simulink model "UUV_Nonlinear_Dynamic_Inversion"  (R2019b)
settings: Solver=ode45  StartTime=0.0  StopTime=600  RelTol=1e-3
undefined symbols (not defined in the file): Amp, Freq
libraries: simulink x4
settings Model: Creator=7385281  LastModifiedBy=7385281
settings SolverCC: AlgebraicLoopSolver=LineSearch

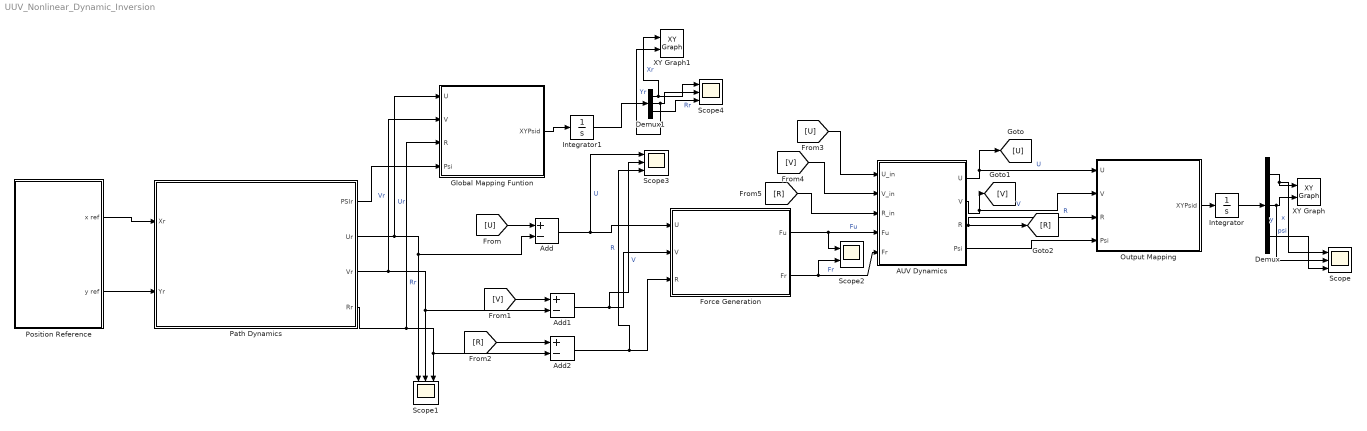
== system UUV_Nonlinear_Dynamic_Inversion ==
  AUV Dynamics : Subsystem
  Add : Sum  Inputs=+-
  Add1 : Sum  Inputs=+-
  Add2 : Sum  Inputs=+-
  Demux : Demux  Outputs=3
  Demux1 : Demux  Outputs=3
  Force Generation : Subsystem
  Global Mapping Funtion : MATLAB Function  TreatAsAtomicUnit=on
  Integrator : Integrator
  Integrator1 : Integrator
  Output Mapping : MATLAB Function  TreatAsAtomicUnit=on
  Path Dynamics : Subsystem
  Position Reference : Subsystem
  Scope{,1,3..4} (4 alike) : Scope  NumInputPorts=3
  Scope2 : Scope  NumInputPorts=2
  XY Graph : simulink/Sinks/XY Graph  xmin=-15  xmax=15  ymin=-15  ymax=15  st=-1
  XY Graph1 : simulink/Sinks/XY Graph  xmin=-15  xmax=15  ymin=-15  ymax=15  st=-1
  wires:
  Position Reference/1(x ref) -> Path Dynamics/1(Xr)
  Position Reference/2(y ref) -> Path Dynamics/2(Yr)
  Force Generation/1(Fu) -> AUV Dynamics/4(Fu), Scope2/1  "Fu"
  Force Generation/2(Fr) -> Scope2/2, AUV Dynamics/5(Fr)  "Fr"
  Path Dynamics/3(Vr) -> Global Mapping Funtion/2(V), Add1/2, Scope1/2  "Vr"
  Path Dynamics/4(Rr) -> Global Mapping Funtion/3(R), Add2/2, Scope1/3  "Rr"
  AUV Dynamics/2(V) -> Output Mapping/2(V), [V]  "V"
  AUV Dynamics/1(U) -> Output Mapping/1(U), [U]  "U"
  AUV Dynamics/3(R) -> [R], Output Mapping/3(R)  "R"
  Path Dynamics/2(Ur) -> Global Mapping Funtion/1(U), Add/2, Scope1/1  "Ur"
  [U] -> Add/1
  Add/1 -> Scope3/1, Force Generation/1(U)  "U"
  [V] -> Add1/1
  [R] -> Add2/1
  Add1/1 -> Scope3/2, Force Generation/2(V)  "V"
  Add2/1 -> Scope3/3, Force Generation/3(R)  "R"
  AUV Dynamics/4(Psi) -> Output Mapping/4(Psi)
  Output Mapping/1(XYPsid) -> Integrator/1
  Demux/1 -> Scope/1, XY Graph/1  "x"
  Demux/2 -> Scope/2, XY Graph/2  "y"
  Integrator/1 -> Demux/1
  Demux/3 -> Scope/3  "psi"
  Path Dynamics/1(PSIr) -> Global Mapping Funtion/4(Psi)
  Global Mapping Funtion/1(XYPsid) -> Integrator1/1
  Integrator1/1 -> Demux1/1
  Demux1/3 -> Scope4/3  "Rr"
  Demux1/2 -> XY Graph1/2, Scope4/2  "Yr"
  Demux1/1 -> XY Graph1/1, Scope4/1  "Xr"
  [U] -> AUV Dynamics/1(U_in)
  [V] -> AUV Dynamics/2(V_in)
  [R] -> AUV Dynamics/3(R_in)

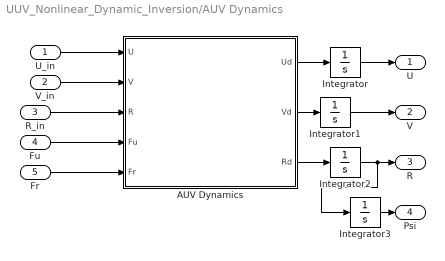
== system UUV_Nonlinear_Dynamic_Inversion/AUV Dynamics ==
  U_in : Inport
  V_in : Inport  Port=2
  R_in : Inport  Port=3
  Fu : Inport  Port=4
  Fr : Inport  Port=5
  AUV Dynamics : MATLAB Function  TreatAsAtomicUnit=on
  Integrator{,1..3} (4 alike) : Integrator
  U : Outport
  V : Outport  Port=2
  R : Outport  Port=3
  Psi : Outport  Port=4
  wires:
  Fr/1 -> AUV Dynamics/5(Fr)
  V_in/1 -> AUV Dynamics/2(V)
  U_in/1 -> AUV Dynamics/1(U)
  R_in/1 -> AUV Dynamics/3(R)
  Fu/1 -> AUV Dynamics/4(Fu)
  Integrator/1 -> U/1
  AUV Dynamics/1(Ud) -> Integrator/1
  AUV Dynamics/2(Vd) -> Integrator1/1
  Integrator1/1 -> V/1
  AUV Dynamics/3(Rd) -> Integrator2/1
  Integrator2/1 -> Integrator3/1, R/1
  Integrator3/1 -> Psi/1

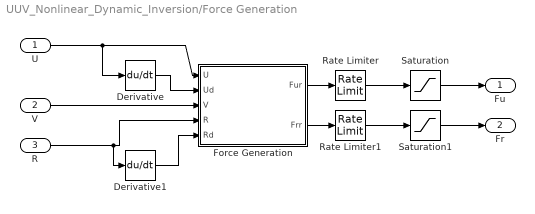
== system UUV_Nonlinear_Dynamic_Inversion/Force Generation ==
  U : Inport
  V : Inport  Port=2
  R : Inport  Port=3
  Derivative : Derivative
  Derivative1 : Derivative
  Force Generation : MATLAB Function  TreatAsAtomicUnit=on
  Rate Limiter : RateLimiter  RisingSlewLimit=50  FallingSlewLimit=-50  SampleTimeMode=inherited
  Rate Limiter1 : RateLimiter  RisingSlewLimit=50  FallingSlewLimit=-50  SampleTimeMode=inherited
  Saturation : Saturate  UpperLimit=50  LowerLimit=-50
  Saturation1 : Saturate  UpperLimit=50  LowerLimit=-50
  Fu : Outport
  Fr : Outport  Port=2
  wires:
  Force Generation/2(Frr) -> Rate Limiter1/1
  R/1 -> Derivative1/1, Force Generation/4(R)
  Derivative1/1 -> Force Generation/5(Rd)
  U/1 -> Force Generation/1(U), Derivative/1
  Force Generation/1(Fur) -> Rate Limiter/1
  V/1 -> Force Generation/3(V)
  Derivative/1 -> Force Generation/2(Ud)
  Rate Limiter/1 -> Saturation/1
  Rate Limiter1/1 -> Saturation1/1
  Saturation/1 -> Fu/1
  Saturation1/1 -> Fr/1

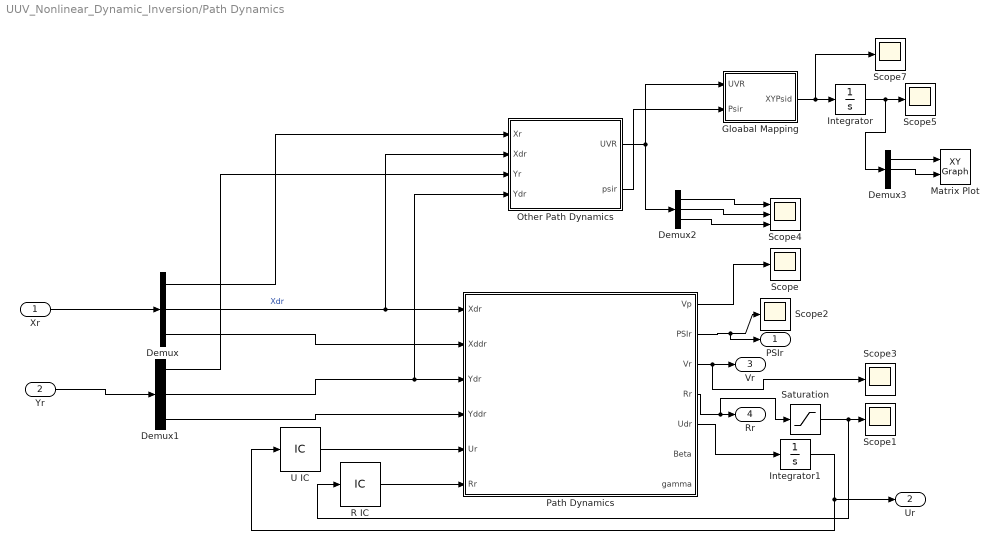
== system UUV_Nonlinear_Dynamic_Inversion/Path Dynamics ==
  Xr : Inport
  Yr : Inport  Port=2
  Demux{,1..3} (4 alike) : Demux  Outputs=3
  Gloabal Mapping : MATLAB Function  TreatAsAtomicUnit=on
  Integrator : Integrator
  Integrator1 : Integrator
  Matrix Plot : simulink/Sinks/XY Graph  xmin=-1  xmax=1  ymin=-1  ymax=1  st=-1
  Other Path Dynamics : MATLAB Function  TreatAsAtomicUnit=on
  Path Dynamics : MATLAB Function  TreatAsAtomicUnit=on
  R IC : InitialCondition  Value=0.001
  Saturation : Saturate
  Scope{,1..3,5,7} (6 alike) : Scope
  Scope4 : Scope  NumInputPorts=3
  U IC : InitialCondition  Value=0.001
  PSIr : Outport
  Ur : Outport  Port=2
  Vr : Outport  Port=3
  Rr : Outport  Port=4
  wires:
  Demux/2 -> Other Path Dynamics/2(Xdr), Path Dynamics/1(Xdr)  "Xdr"
  Path Dynamics/3(Vr) -> Scope3/1, Vr/1
  Xr/1 -> Demux/1
  Path Dynamics/4(Rr) -> Saturation/1, Rr/1
  Path Dynamics/1(Vp) -> Scope/1
  Path Dynamics/2(PSIr) -> PSIr/1, Scope2/1
  Demux/3 -> Path Dynamics/2(Xddr)
  Yr/1 -> Demux1/1
  Demux1/2 -> Other Path Dynamics/4(Ydr), Path Dynamics/3(Ydr)
  Demux1/3 -> Path Dynamics/4(Yddr)
  Demux/1 -> Other Path Dynamics/1(Xr)
  Demux1/1 -> Other Path Dynamics/3(Yr)
  Demux2/1 -> Scope4/1
  Demux2/2 -> Scope4/2
  Demux2/3 -> Scope4/3
  Other Path Dynamics/1(UVR) -> Demux2/1, Gloabal Mapping/1(UVR)
  Other Path Dynamics/2(psir) -> Gloabal Mapping/2(Psir)
  Gloabal Mapping/1(XYPsid) -> Scope7/1, Integrator/1
  Integrator/1 -> Demux3/1, Scope5/1
  Demux3/1 -> Matrix Plot/1
  Demux3/2 -> Matrix Plot/2
  Saturation/1 -> R IC/1, Scope1/1
  U IC/1 -> Path Dynamics/5(Ur)
  Path Dynamics/5(Udr) -> Integrator1/1
  Integrator1/1 -> U IC/1, Ur/1
  R IC/1 -> Path Dynamics/6("Rr ")

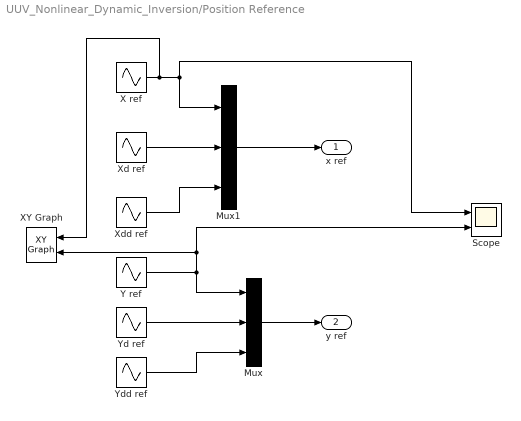
== system UUV_Nonlinear_Dynamic_Inversion/Position Reference ==
  Mux : Mux  Inputs=3
  Mux1 : Mux  Inputs=3
  Scope : Scope  NumInputPorts=2
  X ref : Sin  Amplitude=Amp  Frequency=Freq  SampleTime=0
  XY Graph : simulink/Sinks/XY Graph  xmin=-15  xmax=15  ymin=-15  ymax=15  st=-1
  Xd ref : Sin  Amplitude=Amp*Freq  Frequency=Freq  Phase=pi()/2  SampleTime=0
  Xdd ref : Sin  Amplitude=-Amp*Freq^2  Frequency=Freq  SampleTime=0
  Y ref : Sin  Amplitude=Amp  Frequency=Freq  Phase=pi()/2  SampleTime=0
  Yd ref : Sin  Amplitude=-Amp*Freq  Frequency=Freq  SampleTime=0
  Ydd ref : Sin  Amplitude=-Amp*Freq^2  Frequency=Freq  Phase=pi()/2  SampleTime=0
  x ref : Outport
  y ref : Outport  Port=2
  wires:
  Yd ref/1 -> Mux/2
  Y ref/1 -> Scope/2, XY Graph/2, Mux/1
  Ydd ref/1 -> Mux/3
  Xd ref/1 -> Mux1/2
  Xdd ref/1 -> Mux1/3
  Mux1/1 -> x ref/1
  Mux/1 -> y ref/1
  X ref/1 -> XY Graph/1, Mux1/1, Scope/1

== matlab function UUV_Nonlinear_Dynamic_Inversion/Force Generation/Force Generation ==
  data: U input; Fur output; Ud input; V input; R input; Rd input; Frr output
function [Fur,Frr] = fcn(U,Ud,V,R,Rd)
% This function generates the input forces/torques acting on the AUV
%%%%%%%%%%%%%%%%%%%%%%%%%%%%%%%%%%%%%%%%%%%%%%%%%%%%%%%%%%%%%%%%%%%%%%%%%
% Inputs:
    % U - surge velocity of UUV
    % Ud - derevative of surge velocity
    % V - sway velocity of UUV
    % R- yaw velocity of UUV
    % Rd - derivative of yaw velocity of UUV
% Outputs:
    % Fur - reference surge thrust
    % Frr - reference yaw toque
% Constants:
m1 = 215; % mass (added+rigid) [kg]
m2 = 265; % mass (added+rigid) [kg]
m3 = 80; % inertia (added+rigid) [kg*m^2]

Xu = 70; % Surge Linear Drag [kg/s]
Xuu = 100; % Surge Quadratic Drag [kg/s]

Yv = 100; % Sway Linear Drag [kg/s]
Yvv = 200; % Sway Quadratic Drag [kg/m]

Nr = 50; % Yaw Linear Drag [kg*m^2/s]
Nrr = 100; % Yaw Quadratic Drag [kg*m^2]
%%%%%%%%%%%%%%%%%%%%%%%%%%%%%%%%%%%%%%%%%%%%%%%%%%%%%%%%%%%%%%%%%%%%%%%%%%
% Main Code:
% Force [N]
Fur = m1*Ud-m2*V*R+Xu*U+Xuu*U^2;
Frr = m3*Rd + (m2-m1)*U*V+Nr*R-Nrr*R;

== matlab function UUV_Nonlinear_Dynamic_Inversion/Path Dynamics/Path Dynamics ==
  data: Vp output; Xdr input; Xddr input; PSIr output; Ydr input; Yddr input; Vr output; Rr output; Udr output; Ur input; Beta output; gamma output; Rr input
function [Vp,PSIr,Vr,Rr,Udr,Beta,gamma] = fcn(Xdr,Xddr,Ydr,Yddr,Ur,Rr)
% Function calculates the desired U,V, and R corresponding to the input
% reference X, Y
%%%%%%%%%%%%%%%%%%%%%%%%%%%%%%%%%%%%%%%%%%%%%%%%%%%%%%%%%%%%%%%%%%%%%%%%%%
% Inputs:
    % Xdr - reference x velocity
    % Xddr - refernce x acceleration
    % Ydr - reference y velocity
    % Yddr - reference y acceleration
    % Ur - reference surge velocity
    % Rr - reference yaw velocity
%%%%%%%%%%%%%%%%%%%%%%%%%%%%%%%%%%%%%%%%%%%%%%%%%%%%%%%%%%%%%%%%%%%%%%%%%%
% Outputs:
    % Vp - resultant velocity
    % PSIr- generated psi reference
    % Vr - generated sway reference velocity
    % Rr - generated yaw reference velocity
    % Urd - generated surge derivative reference
    % Beta - angle reference used for debugging
    % Gamma - angle reference used for debugging
%%%%%%%%%%%%%%%%%%%%%%%%%%%%%%%%%%%%%%%%%%%%%%%%%%%%%%%%%%%%%%%%%%%%%%%%%%
% Constants:
m1 = 215; % mass (added+rigid) [kg]
m2 = 265; % mass (added+rigid) [kg]
m3 = 80; % inertia (added+rigid) [kg*m^2]

Xu = 70; % Surge Linear Drag [kg/s]
Xuu = 100; % Surge Quadratic Drag [kg/s]

Yv = 100; % Sway Linear Drag [kg/s]
Yvv = 200; % Sway Quadratic Drag [kg/m]

Nr = 50; % Yaw Linear Drag [kg*m^2/s]
Nrr = 100; % Yaw Quadratic Drag [kg*m^2]
%%%%%%%%%%%%%%%%%%%%%%%%%%%%%%%%%%%%%%%%%%%%%%%%%%%%%%%%%%%%%%%%%%%%%%%%%%%
% Main Code:
% Tangent Velocity to path
Vp = sqrt(Xdr^2+Ydr^2);

% Derivative of tangent path velocity

    Vpd = (Xdr*Xddr+Ydr*Yddr)/Vp;
    
% Reference Sway Velocity
Vr = sqrt(abs(Vp^2-Ur^2));

% Calculate Reference Surge Velocity derivative ( Body forward Velocity)
Udr = ((m1-m2)*Ur*Vp^3)^-1;
% For CCW Rotation
if (Vr < 0) && (Rr > 0)
    Udr = Udr*(-(Vp^3)*(m2*Vp*Vpd+Yv*(Vp^2-Ur^2))+m1*Ur*(Ur*Vpd*Vp^2 + Vp*sqrt(Vp^2-Ur^2 * (Xddr*Ydr-Xdr*Yddr)))- Yvv*(Vp^2-Ur^2)*Vp^3 * sqrt(Vp^2-Ur^2));

% CW Rotation
else
    Udr = Udr*(-(Vp^3)*(m2*Vp*Vpd+Yv*(Vp^2-Ur^2))+m1*(Ur*Vpd*Vp^2 + Vp*sqrt(Vp^2-Ur^2 * (Xddr*Ydr-Xdr*Yddr)))- Yvv*(Vp^2-Ur^2)*Vp^3 * sqrt(Vp^2-Ur^2));
end

% Direction of Vp,
    Beta = atan2(Ydr,Xdr);

% Derivative of Beta
    omega = (Xdr*Yddr-Ydr*Xddr)/(Xdr^2+Ydr^2);



% Calculates gamma angle
 gamma = -atan2(Vr,Ur);
 
% PSI represents the angle between the inertial x axis and the body x axis
PSIr = atan2(Ydr,Xdr)-atan2(Vr,Ur);

% Debugging Lines ( Can be deleted later)
G = Vp*Vr;
Q = Ur*Vpd-Udr*Vp;

% Reference Yaw Velocity ( Angular Velocity about z-axis)
    Rr = omega - (Ur*Vpd-Udr*Vp)/(Vp*Vr);

== matlab function UUV_Nonlinear_Dynamic_Inversion/AUV Dynamics/AUV Dynamics ==
  data: U input; Ud output; V input; R input; Fu input; Fr input; Vd output; Rd output
function [Ud,Vd,Rd] = fcn(U,V,R,Fu,Fr)
% Function models the dynamics of the UUV and its response to the force
% inputs
%%%%%%%%%%%%%%%%%%%%%%%%%%%%%%%%%%%%%%%%%%%%%%%%%%%%%%%%%%%%%%%%%%%%%%%%
% Inputs:
    % U - surge velocity of UUV
    % V - sway velocity of UUV
    % R - yaw velocity of UUV
    % Fu - surge force input
    % Fr - yaw toque input
% Outputs:
    % Ud - derivative of surge velocity
    % Vd - derivitive of sway velocity
    % Rd - derivative of yaw velocity

%%%%%%%%%%%%%%%%%%%%%%%%%%%%%%%%%%%%%%%%%%%%%%%%%%%%%%%%%%%%%%%%%%%%%%%%%%
% Constants
m1 = 215; % mass (added+rigid) [kg]
m2 = 265; % mass (added+rigid) [kg]
m3 = 80; % inertia (added+rigid) [kg*m^2]

Xu = 70; % Surge Linear Drag [kg/s]
Xuu = 100; % Surge Quadratic Drag [kg/s]

Yv = 100; % Sway Linear Drag [kg/s]
Yvv = 200; % Sway Quadratic Drag [kg/m]

Nr = 50; % Yaw Linear Drag [kg*m^2/s]
Nrr = 100; % Yaw Quadratic Drag [kg*m^2]
%%%%%%%%%%%%%%%%%%%%%%%%%%%%%%%%%%%%%%%%%%%%%%%%%%%%%%%%%%%%%%%%%%%%%%%%%%%
% Main Code:

% AUV dynamics, outputs the derivate of U, V, and R
Ud = V*R*m2/m1 - Xu*U/m1 - Xuu*U*abs(U)/m1+Fu/m1;
Vd = -m1*U*R/m2 - Yv*V/m2 - Yvv*V*abs(V);
Rd = (m1-m2)*U*V/m3 - Nr*R/m3 - Nrr/m3 + Fr/m3;

== matlab function UUV_Nonlinear_Dynamic_Inversion/Output Mapping ==
  data: U input; V input; R input; Psi input; XYPsid output
function XYPsid = fcn(U,V,R,Psi)
% Funtion maps the body fixed velocities to the world-fixed velocities
%Inputs: U,V,R - surge,sway, yaw velocities of UUV
    % Psi - orientation of UUV about z axis
% Outputs:
    %XYPsid - 3x1 vector of the world-fixed velocities
 %%%%%%%%%%%%%%%%%%%%%%%%%%%%%%%%%%%%%%%%%%%%%%%%%%%%%%%%%%%%%%%%%%%%%%%
 % Mapping
A = [cos(Psi) -sin(Psi) 0; sin(Psi) cos(Psi) 0; 0 0 1];
Q = [U; V; R];
XYPsid = A*Q;

== matlab function UUV_Nonlinear_Dynamic_Inversion/Global Mapping Funtion ==
  data: U input; V input; R input; Psi input; XYPsid output
function XYPsid = fcn(U,V,R,Psi)
% Debugging funtion
% Transform back to X, Y to check if path dynamics is outputing correctly

A = [cos(Psi) -sin(Psi) 0; sin(Psi) cos(Psi) 0; 0 0 1];
Q = [U; V; R];
XYPsid = A*Q;

== matlab function UUV_Nonlinear_Dynamic_Inversion/Path Dynamics/Other Path Dynamics ==
  data: Xr input; UVR output; Xdr input; Yr input; Ydr input; psir output
function [UVR,psir] = fcn(Xr,Xdr,Yr,Ydr)
% Transform from Global/inertial to body coordinate system
% DEbugging funtion
% Trying to figure out if this is a better method

% Calculate reference psi
psir = atan(Yr/Xr);

% Calculates derivative of ref psi
    % Not entirely sure about these "inputs"
psidr = 1/(1+psir^2);

% Transformation matrices
B = [Xdr; Ydr; psidr];
A = [cos(psir) -sin(psir) 0; sin(psir) cos(psir) 0; 0 0 1];
UVR = A\B;

== matlab function UUV_Nonlinear_Dynamic_Inversion/Path Dynamics/Gloabal Mapping ==
  data: UVR input; XYPsid output; Psir input
function XYPsid = fcn(UVR,Psir)
% Transforming back into x, y for debuging to check if method works

A = [cos(Psir) -sin(Psir) 0; sin(Psir) cos(Psir) 0; 0 0 1];
XYPsid = A*UVR;
